simulink model "controller"  (R2022b)
settings: Solver=VariableStepAuto  StartTime=0.0  StopTime=50.2  RelTol=1e-3
settings Model: Creator=me-clab2  LastModifiedBy=X1
settings SolverCC: AlgebraicLoopSolver=TrustRegion
settings DebuggingCC: UnconnectedInputMsg=warning  UnconnectedOutputMsg=warning  UnconnectedLineMsg=warning  SFMachineParentedDataDiag=warning
settings ModelReferenceCC: EnableRefExpFcnMdlSchedulingChecks=on

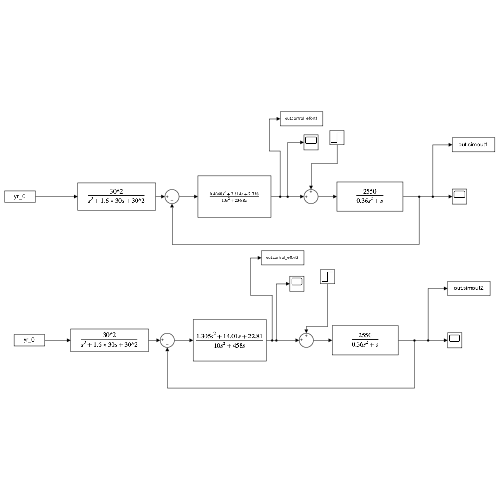
[thumbnail: Simulink's stored preview of the top-level diagram]
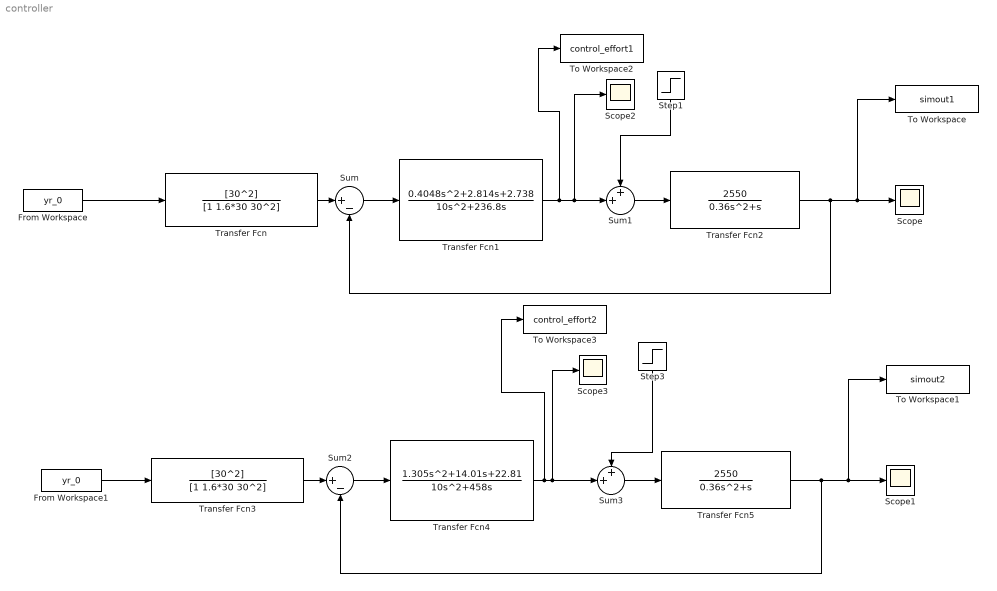
== system controller ==
  From Workspace : FromWorkspace  VariableName=yr_0
  From Workspace1 : FromWorkspace  VariableName=yr_0
  Scope{,1..3} (4 alike) : Scope
  Step1 : Step  Time=0  After=0  SampleTime=0
  Step3 : Step  Time=0  After=0  SampleTime=0
  Sum : Sum  Inputs=|+-
  Sum1 : Sum  Inputs=++|
  Sum2 : Sum  Inputs=|+-
  Sum3 : Sum  Inputs=++|
  To Workspace : ToWorkspace  VariableName=simout1  SaveFormat=Timeseries  SampleTime=-1
  To Workspace1 : ToWorkspace  VariableName=simout2  SaveFormat=Timeseries  SampleTime=-1
  To Workspace2 : ToWorkspace  VariableName=control_effort1  SaveFormat=Timeseries  SampleTime=-1
  To Workspace3 : ToWorkspace  VariableName=control_effort2  SaveFormat=Timeseries  SampleTime=-1
  Transfer Fcn : TransferFcn  Numerator=[30^2]  Denominator=[1 1.6*30 30^2]
  Transfer Fcn1 : TransferFcn  Numerator=[0.4048 2.814 2.738]  Denominator=[10 236.8 0]
  Transfer Fcn2 : TransferFcn  Numerator=[2550]  Denominator=[0.36 1 0]
  Transfer Fcn3 : TransferFcn  Numerator=[30^2]  Denominator=[1 1.6*30 30^2]
  Transfer Fcn4 : TransferFcn  Numerator=[1.305 14.01 22.81]  Denominator=[10 458 0]
  Transfer Fcn5 : TransferFcn  Numerator=[2550]  Denominator=[0.36 1 0]
  wires:
  Transfer Fcn/1 -> Sum/1
  Sum/1 -> Transfer Fcn1/1
  Transfer Fcn1/1 -> To Workspace2/1, Scope2/1, Sum1/2
  Sum1/1 -> Transfer Fcn2/1
  Transfer Fcn2/1 -> Sum/2, To Workspace/1, Scope/1
  From Workspace/1 -> Transfer Fcn/1
  Step1/1 -> Sum1/1
  Step3/1 -> Sum3/1
  From Workspace1/1 -> Transfer Fcn3/1
  Transfer Fcn3/1 -> Sum2/1
  Sum3/1 -> Transfer Fcn5/1
  Transfer Fcn4/1 -> To Workspace3/1, Scope3/1, Sum3/2
  Sum2/1 -> Transfer Fcn4/1
  Transfer Fcn5/1 -> Sum2/2, To Workspace1/1, Scope1/1
